simulink model "constraints_comparison_A_4D_v2_old"  (R2016a)
settings: Solver=ode4  StartTime=0.0  StopTime=10  FixedStep=0.0001  RelTol=1e-3
InitFcn:
  | clear
  | clc
undefined symbols (not defined in the file or in its folder): acm_aero_model, acm_T_N, breakpoints1, Cm0, Cmde, Cmq, dail, de, dele, drud, Fr_mp_1, Fr_mp_2, Fr_rp_1, Fr_rp_2, ini_acm_de_deg, ini_acm_p_deg_per_s, ini_acm_phi_deg, ini_acm_psi_deg, ini_acm_q_deg_per_s, ini_acm_r_deg_per_s, ini_acm_theta_deg, ini_cmp_de_deg, ini_rig_p_deg_per_s, ini_rig_phi_deg, ini_rig_psi_deg, ini_rig_q_deg_per_s, ini_rig_r_deg_per_s, ini_rig_theta_deg, K1_svo_acm, K1_svo_cmp, K2_svo_acm, K2_svo_cmp, La, Ma, max_defl_sat_acm, max_defl_sat_cmp, max_rate_sat, max_rate_sat_acm, max_rate_sat_cmp, Na, sigbuilder_block, simstop, windspeed, Xa, Ya, Za
libraries: aerolibconvert2 x117, simulink x42, aerolibtransform2 x19, vrlib x2
(part 2 of 6)

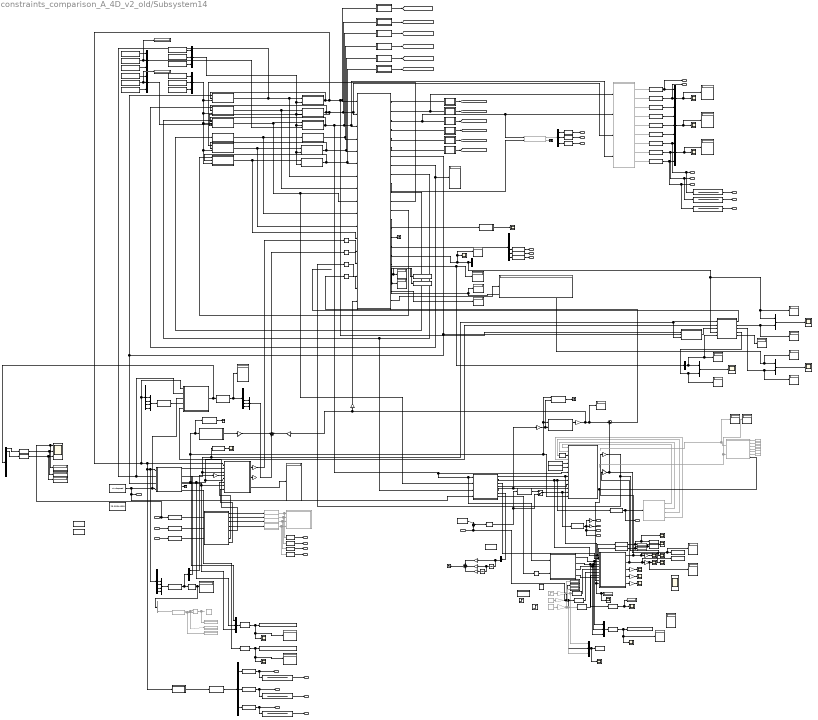
== system constraints_comparison_A_4D_v2_old/Subsystem14 ==
  note: yaw
  note: pitch
  note: roll
  note: Estimated reaction forces
  note: Simulation aircraft reaction forces
  note: Estimated laod cell reading
  note: Simulation load cell reading
  note: ALTITUDE CONTROL
  note: Estimated estimated load cell moment
  note: Simulation load cell moment
  ACM_de_c(deg) : Inport
  CMP_da_c(deg) : Inport  Port=2
  CMP_de_c(deg) : Inport  Port=3
  CMP_dr_c(deg) : Inport  Port=4
  Aerodynamics lookup : Subsystem  Commented=on
  Aerodynamics model: Hawk : MATLAB Function
      settings: MinAlgLoopOccurrences=on
  Aerodynamics model: compensator : MATLAB Function
      settings: MinAlgLoopOccurrences=on
  Aircraft acceleration body axis : MATLAB Function  Commented=on  TreatAsAtomicUnit=on
  Aircraft attitude relative to arm2 : MATLAB Function  Commented=on  TreatAsAtomicUnit=on
  Aircraft loads for load case loop : MATLAB Function  Commented=on
      settings: MinAlgLoopOccurrences=on
  Aircraft model vertical reaction force : Scope
  Aircraft_model_friction : MATLAB Function
      settings: MinAlgLoopOccurrences=on
  Angle Conversion{,1,3,6,8..12,14..26,29..34,37..38,40} (31 alike) : aerolibconvert2/Angle Conversion  IU=rad  OU=deg
  Angle Conversion{2,4,7,13,27..28,35,39} (8 alike) : aerolibconvert2/Angle Conversion  IU=deg  OU=rad
  Butterworth filter (cutoff frequency 10Hz) + differentiating{,1..5} (6 alike) : TransferFcn  Numerator=[1 0]  Denominator=[2.5330e-04 0.0225 1]
  CMP aero model : MATLABFcn  MATLABFcn=Cmp_aero_model
  Calculating rig pitch acceleration : MATLAB Function  TreatAsAtomicUnit=on
  Chirp Signal : simulink/Sources/Chirp Signal  Commented=on  f1=0.5  T=120  f2=3
  Chirp Signal1 : simulink/Sources/Chirp Signal  Commented=on  f1=0.5  T=120  f2=3
  Chirp Signal2 : simulink/Sources/Chirp Signal  f1=0.5  T=120  f2=3
  Comparing simulation aircraft reaction forces and estimated reaction forces : Scope
  Comparing simulation aircraft reaction forces and estimated reaction forces1 : Scope
  Comparing simulation load cell reading and estimated load cell reading : Scope
  Compensator friction : MATLAB Function
      settings: MinAlgLoopOccurrences=on
  Compensator servo model1 : Subsystem  Commented=on
  Compensator servo model2 : Subsystem  Commented=on
  Compensator servo model3 : Subsystem  Commented=on
  Compensator servo model4 : Subsystem  Commented=on
  Constant : Constant  Commented=on  Value=simstop
  Constant10 : Constant  Value=7.515637662
  Constant11 : Constant  Value=0
  Constant2 : Constant  Value=-7.308232274
  Constant3 : Constant  Value=14.34612797
  Cq_transpose_lc CHECK : Display
  Demux : Demux  Outputs=7
  Demux{1..3,5..6,12} (6 alike) : Demux  Outputs=3
  Demux10 : Demux  Outputs=11
  Demux4 : Demux  Commented=on  Outputs=3
  Demux7 : Demux  Outputs=6
  Demux8 : Demux  Outputs=7
  Demux9 : Demux  Outputs=6
  Derivative : Derivative
  Display{,2..3,5..6,8..14,18} (13 alike) : Display
  Display15 : Display  Commented=on
  Display16 : Display  Commented=on
  Display17 : Display  Commented=on
  Equations of Motion : MATLAB Function
      settings: MinAlgLoopOccurrences=on
  Extracting aircraft vertical reaction forces1 : MATLAB Function  TreatAsAtomicUnit=on
  Extracting position vector 1 : Subsystem
  Extracting position vector 2 : Subsystem
  "Extracting position vector 2 " : Subsystem
  Extracting position vector 3 : Subsystem
  Extracting position vector 4 : Subsystem
  Extracting position vector 5 : Subsystem
  F : Display
  FF : Display
  Fcn : Fcn  Expr=u/9.81
  Fcn1 : Fcn  Expr=u/9.81
  Fcn2 : Fcn  Expr=u/9.81
  Friction_estimate : Display
  Friction_moment : Display
  Gain{,3,6..7,11,14,28} (7 alike) : Gain  Gain=-1
  Gain{4,8..10,17,19..23,30} (11 alike) : Gain
  Gain12 : Gain  Gain=0
  Gain13 : Gain  Gain=0
  Gain24 : Gain  Commented=on  Gain=dail
  Gain25 : Gain  Commented=on  Gain=dele
  Gain27 : Gain  Commented=on  Gain=drud
  HHIRM : MATLAB Function
      settings: MinAlgLoopOccurrences=on
  Hawk servo model : Subsystem
  IC{1..4} (4 alike) : InitialCondition  Value=0
  Integrator : Integrator
  Integrator1 : Integrator
  L : Constant  Commented=on  Value=La
  Load cell reading to aircraft reaction forces : MATLAB Function  TreatAsAtomicUnit=on
  M : Display
  M1 : Constant  Commented=on  Value=Ma
  MATLAB Function1 : MATLAB Function  TreatAsAtomicUnit=on
  MATLAB Function10 : MATLAB Function  TreatAsAtomicUnit=on
  MATLAB Function2 : MATLAB Function  TreatAsAtomicUnit=on
  MATLAB Function3 : MATLAB Function
      settings: MinAlgLoopOccurrences=on
  MATLAB Function4 : MATLAB Function  TreatAsAtomicUnit=on
  MATLAB Function5 : MATLAB Function
      settings: MinAlgLoopOccurrences=on
  MATLAB Function6 : MATLAB Function  TreatAsAtomicUnit=on
  MATLAB Function7 : MATLAB Function
      settings: MinAlgLoopOccurrences=on
  MATLAB Function8 : MATLAB Function  TreatAsAtomicUnit=on
  MATLAB Function9 : MATLAB Function  TreatAsAtomicUnit=on
  MM : Display
  Manual Switch1 : ManualSwitch  CurrentSetting=0
  Mux{,2..4,7..10,12..13,15} (11 alike) : Mux  Inputs=3
  Mux1 : Mux  Inputs=2
  Mux11 : Mux
  Mux14 : Mux
  Mux5 : Mux  Inputs=2
  Mux6 : Mux  Inputs=2
  N : Constant  Commented=on  Value=Na
  Physical deflections to virtual compensator deflections : MATLAB Function  Commented=on  TreatAsAtomicUnit=on
  Quaternions to Rotation Angles : aerolibtransform2/Quaternions to Rotation Angles  rotationOrder=ZYX
  Quaternions to Rotation Angles1 : aerolibtransform2/Quaternions to Rotation Angles  rotationOrder=ZYX
  Quaternions to Rotation Angles2 : aerolibtransform2/Quaternions to Rotation Angles  rotationOrder=ZYX
  Relational Operator : RelationalOperator  Commented=on  OutDataTypeStr=boolean
  Relative angle from rotation matrix : Scope
  Rotation angles from rotation matrix (acm) : Scope
  Rotation angles from rotation matrix (arm) : Scope
  Scope{,1..8,10..13} (13 alike) : Scope
  Scope14 : Scope  NumInputPorts=3
  Scope9 : Scope  NumInputPorts=5
  Signal Builder : Subsystem  Tag=STV Subsys  LoadFcn=sigbuilder_block('load');  StartFcn=sigbuilder_block('start');  StopFcn=sigbuilder_block('stop');  ClipboardFcn=sigbuilder_block('clipboard');  mask(Sigbuilder block){}
      mask help: Simulink:masks:SigbuilderBlock_MD
      mask init:
      | if ~strcmp(get_param(bdroot(gcbh),'SimulationStatus'),'stopped') tuvar = sigbuilder_block('maskInit'); end
      settings: CopyFcn=sigbuilder_block('copy');  DeleteFcn=sigbuilder_block('delete');  ModelCloseFcn=sigbuilder_block('modelClose');  PreSaveFcn=sigbuilder_block('preSave');  PauseFcn=sigbuilder_block('pause');  ContinueFcn=sigbuilder_block('continue');  NameChangeFcn=sigbuilder_block('namechange');  OpenFcn=sigbuilder_block('open',[437.6 199.2 550.4 400 ]);  CloseFcn=sigbuilder_block('close');
      mask Display: plot(0, 0, 100, 100,[2, 2, 32, 32, 2], [68, 8, 8, 68, 68],[32, 2], [38, 38], [32, 19, 2],[53, 60, 44], [32, 17, 17, 2],[16, 16, 31, 31]);txt = getActiveGroup(gcbh);text(2, 100, txt,'verticalAlignment', 'top');
  Step : Step  Commented=on  Time=0.01  SampleTime=0
  Step2 : Step  SampleTime=0
  Step3 : Step  SampleTime=0
  Stop Simulation : Stop  Commented=on
  Subsystem : Subsystem
  Subsystem1 : Subsystem
  Subsystem10 : Subsystem
  Subsystem11 : Subsystem
  Subsystem12 : Subsystem
  Subsystem13 : Subsystem
  Subsystem2 : Subsystem
  Subsystem3 : Subsystem
  Subsystem4 : Subsystem
  Subsystem5 : Subsystem
  Subsystem6 : Subsystem
  Subsystem7 : Subsystem
  Subsystem8 : Subsystem
  Subsystem9 : Subsystem
  Sum2 : Sum  Inputs=|++
  Sum3 : Sum
  Sum5 : Sum  Inputs=+++
  Sum8 : Sum  Inputs=++-
  Terminator{,1..5} (6 alike) : Terminator
  To Workspace : ToWorkspace  VariableName=reaction_forces_lc_body_N  SaveFormat=Timeseries  SampleTime=-1
  To Workspace1 : ToWorkspace  VariableName=reaction_moments_lc_body_Nm  SaveFormat=Timeseries  SampleTime=-1
  To Workspace2 : ToWorkspace  VariableName=cs_deg  SaveFormat=Timeseries  SampleTime=-1
  To Workspace3 : ToWorkspace  VariableName=alpha_deg  SaveFormat=Timeseries  SampleTime=-1
  To Workspace4 : ToWorkspace  VariableName=beta_deg  SaveFormat=Timeseries  SampleTime=-1
  To Workspace5 : ToWorkspace  VariableName=aero_forces_N  SaveFormat=Timeseries  SampleTime=-1
  To Workspace6 : ToWorkspace  VariableName=aero_moments_Nm  SaveFormat=Timeseries  SampleTime=-1
  To Workspace7 : ToWorkspace  VariableName=wind_axes_rotation_rates_degpers  SaveFormat=Timeseries  SampleTime=-1
  To Workspace8 : ToWorkspace  VariableName=inertial_axes_CMP_rotation_rates_degpers  SaveFormat=Timeseries  SampleTime=-1
  To Workspace9 : ToWorkspace  VariableName=inertial_axes_CMP_rotation_accelerations_degperspers  SaveFormat=Timeseries  SampleTime=-1
  V{,1..3} (4 alike) : Display
  Virtual compensator deflections to physical deflections : MATLAB Function  TreatAsAtomicUnit=on
  Wind axes angular rates calculation : MATLAB Function
      settings: MinAlgLoopOccurrences=on
  Wind tunnel velocity : Constant  Value=windspeed
  Wind tunnel velocity1 : Constant  Value=25.09344509
  X : Constant  Commented=on  Value=Xa
  Y : Constant  Commented=on  Value=Ya
  Z : Constant  Commented=on  Value=Za
  acm_T_N : Constant  Value=acm_T_N
  acm_aero_model : Constant  Value=acm_aero_model
  aircraft_cell_reaction_forces : Display
  aircraft_cell_reaction_moments : Display
  alpha : Display
  alpha1 : Display
  alpha2 : Scope
  beta2 : Scope
  ini_acm_q_deg_per_s : Constant  Value=ini_acm_q_deg_per_s
  ini_acm_q_deg_per_s2 : Constant  Value=ini_acm_p_deg_per_s
  ini_acm_q_deg_per_s3 : Constant  Value=ini_acm_r_deg_per_s
  ini_acm_theta_deg : Constant  Value=ini_acm_theta_deg
  ini_acm_theta_deg2 : Constant  Value=ini_acm_phi_deg
  ini_acm_theta_deg3 : Constant  Value=ini_acm_psi_deg
  ini_rig_theta_deg : Constant  Value=ini_rig_theta_deg
  ini_rig_theta_deg2 : Constant  Value=ini_rig_psi_deg
  ini_rig_theta_deg3 : Constant  Value=ini_rig_phi_deg
  ini_rig_theta_deg_per_s : Constant  Value=ini_rig_q_deg_per_s
  ini_rig_theta_deg_per_s2 : Constant  Value=ini_rig_p_deg_per_s
  ini_rig_theta_deg_per_s3 : Constant  Value=ini_rig_r_deg_per_s
  load_cell_reaction_forces{,2..8} (8 alike) : Display
  load_cell_reaction_forces_body : Display
  load_cell_reaction_moments : Display
  load_cell_reaction_moments_body : Display
  q : Display
  q1 : Display
  rates : Display
  theta_rig : Scope
  z_reaction_force : Scope
  GX(deg/s) : Outport
  GY(deg/s) : Outport  Port=2
  GZ(deg/s) : Outport  Port=3
  Nx : Outport  Port=4
  Ny : Outport  Port=5
  Nz : Outport  Port=6
  ACM_roll(deg) : Outport  Port=7
  ACM_rollrate(deg/s) : Outport  Port=8
  ACM_pitch(deg) : Outport  Port=9
  ACM_pitchrate(deg/s) : Outport  Port=10
  ACM_yaw(deg) : Outport  Port=11
  ACM_yawrate(deg/s) : Outport  Port=12
  RIG_roll(deg) : Outport  Port=13
  RIG_rollrate(deg/s) : Outport  Port=14
  RIG_pitch(deg) : Outport  Port=15
  RIG_pitchrate(deg/s) : Outport  Port=16
  RIG_yaw(deg) : Outport  Port=17
  RIG_yawrate(deg/s) : Outport  Port=18
  delta_el_c(deg) : Outport  Port=19
  delta_el(deg) : Outport  Port=20
  delta_er_c(deg) : Outport  Port=21
  delta_er(deg) : Outport  Port=22
  delta_cmp1(deg) : Outport  Port=23
  delta_cmp2(deg) : Outport  Port=24
  delta_cmp3(deg) : Outport  Port=25
  delta_cmp4(deg) : Outport  Port=26
  wind speed(m/s) : Outport  Port=27
  AoA(deg) : Outport  Port=28
  roll_ac(deg) : Outport  Port=29
  pitch_ac(deg) : Outport  Port=30
  tag scope: animation_acm_rotation=global, animation_acm_translation=global, animation_arm_rotation=global, animation_arm_translation=global, animation_cmp_rotation=global, animation_cmp_translation=global, animation_link_rotation=global, animation_link_translation=global, animation_load_cell_rotation=global, animation_load_cell_translation=global, animation_mass_rotation=global, animation_mass_translation=global
  wires:
  Equations of Motion/2(Ar) -> Aircraft attitude relative to arm2/1(Ar), MATLAB Function1/1(A2)
  Equations of Motion/8(qr_dot_dot) -> Subsystem2/1(In1), load_cell_reaction_forces8/1
  Subsystem2/1(Out1) -> Equations of Motion/8(qr_dot), Subsystem3/1(In1)
  Angle Conversion2/1 -> Hawk servo model/1(Command), Manual Switch1/2
  Sum3/1 -> Angle Conversion2/1  "Hawk elevator (deg)"
  Equations of Motion/11(qm_dot_dot) -> Subsystem8/1(In1)
  Subsystem8/1(Out1) -> Equations of Motion/10(qm_dot), Subsystem9/1(In1)
  Subsystem9/1(Out1) -> Extracting position vector 4/1(In1), Equations of Motion/4(qm)
  Equations of Motion/4(Am) -> MATLAB Function8/1(A3)
  Compensator friction/1(Fr_rp) -> Gain12/1
  Extracting aircraft vertical reaction forces1/1(RF_a) -> Aircraft model vertical reaction force/1
  Gain13/1 -> Friction_moment/1, Sum2/1, Gain30/1, Gain3/1  "Friction moment"
  Gain30/1 -> Sum8/3
  Gain20/1 -> Subsystem6/2(theta_dot_mp), Aircraft_model_friction/2(theta_dot_mp)
  Equations of Motion/14(RF) -> Extracting aircraft vertical reaction forces1/1(RF)
  Angle Conversion1/1 -> AoA(deg)/1, Aerodynamics lookup/1(Alpha (deg))  "Hawk alpha (deg)"
  MATLAB Function4/1(q2) -> Quaternions to Rotation Angles/1
  Quaternions to Rotation Angles/1 -> Demux3/1
  Demux3/2 -> Angle Conversion9/1
  Aircraft acceleration body axis/1(qa_dot_dot3) -> Demux5/1
  Integrator/1 -> Integrator1/1, Gain/1
  Demux6/3 -> Gain7/1, Integrator/1
  Gain/1 -> Sum5/2
  Integrator1/1 -> Gain6/1
  Gain6/1 -> Sum5/3
  Gain7/1 -> Sum5/1
  Demux3/1 -> Angle Conversion8/1
  Butterworth filter (cutoff frequency 10Hz) + differentiating/1 -> RIG_rollrate(deg/s)/1
  Butterworth filter (cutoff frequency 10Hz) + differentiating2/1 -> RIG_yawrate(deg/s)/1
  Demux3/3 -> Angle Conversion10/1
  Angle Conversion8/1 -> RIG_roll(deg)/1, Butterworth filter (cutoff frequency 10Hz) + differentiating/1
  Angle Conversion9/1 -> Butterworth filter (cutoff frequency 10Hz) + differentiating1/1, RIG_pitch(deg)/1
  Angle Conversion10/1 -> RIG_yaw(deg)/1, Butterworth filter (cutoff frequency 10Hz) + differentiating2/1
  Demux5/1 -> Fcn/1
  Demux5/2 -> Fcn1/1
  Demux5/3 -> Fcn2/1
  Equations of Motion/16(qa_dot2) -> Demux7/1
  Demux7/4 -> Angle Conversion/1
  Demux7/5 -> Angle Conversion11/1
  Demux7/6 -> Angle Conversion12/1
  Fcn/1 -> Nx/1
  Fcn1/1 -> Ny/1
  Fcn2/1 -> Nz/1
  Angle Conversion/1 -> GX(deg/s)/1
  Angle Conversion11/1 -> GY(deg/s)/1
  Angle Conversion12/1 -> GZ(deg/s)/1
  Subsystem3/1(Out1) -> Subsystem2/2(q), Subsystem4/5(qr), "Extracting position vector 2 "/1(In1), Equations of Motion/2(qr), Aircraft attitude relative to arm2/3(qr)
  Equations of Motion/3(Aa) -> MATLAB Function6/1(A3), Aircraft acceleration body axis/1(Aa), Aircraft attitude relative to arm2/2(Aa)
  Mux2/1 -> Relative angle from rotation matrix/1, Display/1
  Aircraft attitude relative to arm2/7(phi_relative) -> Angle Conversion16/1
  Aircraft attitude relative to arm2/9(psi_relative) -> Angle Conversion18/1
  Angle Conversion18/1 -> Butterworth filter (cutoff frequency 10Hz) + differentiating5/1, ACM_yaw(deg)/1, Mux2/3  "Yaw"
  Angle Conversion17/1 -> Mux2/2, Butterworth filter (cutoff frequency 10Hz) + differentiating4/1, ACM_pitch(deg)/1  "Pitch"
  Angle Conversion16/1 -> ACM_roll(deg)/1, Butterworth filter (cutoff frequency 10Hz) + differentiating3/1, Mux2/1  "Roll"
  Mux3/1 -> Display2/1, Rotation angles from rotation matrix (acm)/1
  Angle Conversion21/1 -> Mux3/3  "Yaw"
  Angle Conversion20/1 -> pitch_ac(deg)/1, Mux3/2  "Pitch"
  Angle Conversion19/1 -> roll_ac(deg)/1, Mux3/1  "Roll"
  Aircraft attitude relative to arm2/1(phi_acm) -> Angle Conversion19/1
  Aircraft attitude relative to arm2/2(theta_acm) -> Angle Conversion20/1
  Aircraft attitude relative to arm2/3(psi_acm) -> Angle Conversion21/1
  Mux4/1 -> Rotation angles from rotation matrix (arm)/1, Display3/1
  Angle Conversion24/1 -> Mux4/3  "Yaw"
  Angle Conversion23/1 -> Mux4/2  "Pitch"
  Angle Conversion22/1 -> Mux4/1  "Roll"
  Aircraft attitude relative to arm2/4(phi_arm) -> Angle Conversion22/1
  Aircraft attitude relative to arm2/5(theta_arm) -> Angle Conversion23/1
  Aircraft attitude relative to arm2/6(psi_arm) -> Angle Conversion24/1
  Butterworth filter (cutoff frequency 10Hz) + differentiating3/1 -> ACM_rollrate(deg/s)/1
  Butterworth filter (cutoff frequency 10Hz) + differentiating4/1 -> ACM_pitchrate(deg/s)/1
  Butterworth filter (cutoff frequency 10Hz) + differentiating5/1 -> ACM_yawrate(deg/s)/1
  CMP_da_c(deg)/1 -> Display12/1, Scope14/1, Angle Conversion35/1  "input (deg)"
  CMP_dr_c(deg)/1 -> Angle Conversion39/1
  Angle Conversion6/1 -> Gain11/1, Gain14/1, delta_er(deg)/1, delta_er_c(deg)/1
  Virtual compensator deflections to physical deflections/1(servo1) -> Compensator servo model1/1(Command)
  Virtual compensator deflections to physical deflections/2(servo2) -> Compensator servo model2/1(Command)
  Virtual compensator deflections to physical deflections/3(servo3) -> Compensator servo model3/1(Command)
  Virtual compensator deflections to physical deflections/4(servo4) -> Compensator servo model4/1(Command)
  Angle Conversion4/1 -> Aerodynamics model: Hawk/3(de)
  Aerodynamics lookup/1(Cm0) -> Aerodynamics model: Hawk/1(Cm0)
  Aerodynamics lookup/2(Cmde) -> Aerodynamics model: Hawk/2(Cmde)
  Aerodynamics lookup/3(de_deg) -> Angle Conversion4/1
  Aerodynamics lookup/4(Cmq) -> Aerodynamics model: Hawk/4(Cmq)
  Angle Conversion14/1 -> delta_cmp1(deg)/1
  Angle Conversion15/1 -> delta_cmp2(deg)/1
  Angle Conversion25/1 -> delta_cmp3(deg)/1
  Angle Conversion26/1 -> delta_cmp4(deg)/1
  MATLAB Function2/1(A11) -> [animation_cmp_rotation]
  MATLAB Function1/1(A22) -> [animation_arm_rotation]
  MATLAB Function6/1(A33) -> [animation_acm_rotation]
  MATLAB Function8/1(A33) -> [animation_mass_rotation]
  Extracting position vector 1/1(Out1) -> [animation_cmp_translation]
  "Extracting position vector 2 "/1(Out1) -> [animation_arm_translation]
  Extracting position vector 3/1(Out1) -> [animation_acm_translation]
  Extracting position vector 4/1(Out1) -> [animation_mass_translation]
  Compensator servo model1/1(Response) -> Angle Conversion14/1, Physical deflections to virtual compensator deflections/1(servo1)
  Compensator servo model2/1(Response) -> Angle Conversion15/1, Physical deflections to virtual compensator deflections/2(servo2)
  Compensator servo model3/1(Response) -> Angle Conversion25/1, Physical deflections to virtual compensator deflections/3(servo3)
  Compensator servo model4/1(Response) -> Angle Conversion26/1, Physical deflections to virtual compensator deflections/4(servo4)
  Equations of Motion/1(Ac) -> MATLAB Function2/1(A1)
  Manual Switch1/1 -> Angle Conversion6/1, Aerodynamics model: Hawk/12(eta)
  Virtual compensator deflections to physical deflections/7(de_cmp2) -> Aerodynamics model: compensator/6(eta)
  MATLAB Function7/1(V_t) -> Aerodynamics model: compensator/2(V_t)
  MATLAB Function3/1(V0) -> HHIRM/11(V), Scope6/1, V/1, Aerodynamics model: Hawk/8(V0)
  MATLAB Function3/2(alpha) -> Angle Conversion3/1, HHIRM/1(alpha), Angle Conversion1/1, Aerodynamics model: Hawk/9(alpha)
  MATLAB Function3/4(w_dot) -> Aerodynamics model: Hawk/10(w_dot)
  MATLAB Function3/5(q) -> Gain20/1, Aerodynamics model: Hawk/11(q)
  MATLAB Function3/6(Va) -> Demux6/1
  Aerodynamics model: compensator/1(F_c) -> Gain4/1
  Aerodynamics model: compensator/2(M_dash_c) -> Gain8/1
  Gain12/1 -> Sum8/1
  Equations of Motion/10(qa_dot_dot2) -> Aircraft acceleration body axis/2(qa_dot_dot2)
  Aircraft attitude relative to arm2/8(theta_relative) -> Angle Conversion17/1
  Aircraft_model_friction/1(Fr_mp) -> Gain13/1
  Mux15/1 -> Sum8/2
  Hawk servo model/1(Response) -> Manual Switch1/1
  Gain4/1 -> IC1/1
  Sum8/1 -> IC2/1
  Gain10/1 -> Scope5/1, IC3/1
  Sum2/1 -> IC4/1
  Subsystem5/1(Out1) -> Extracting position vector 3/1(In1), Equations of Motion/3(qa), Aircraft attitude relative to arm2/4(qa), Wind axes angular rates calculation/1(qa), MATLAB Function3/1(qa), Aerodynamics model: Hawk/7(qa), Subsystem4/2(qa)
  Subsystem4/1(Out1) -> Subsystem5/1(In1), MATLAB Function3/2(qa_dot), Equations of Motion/9(qa_dot)
  Equations of Motion/9(qa_dot_dot) -> Subsystem4/1(In1), MATLAB Function3/3(qa_dot_dot)
  IC1/1 -> Equations of Motion/13(F_c)
  IC2/1 -> Equations of Motion/14(M_dash_c)
  IC3/1 -> Equations of Motion/15(F_a)
  IC4/1 -> Equations of Motion/16(M_dash_a)
  Mux8/1 -> Subsystem1/2(rig attitude), Subsystem3/2(rig attitude), Subsystem5/2(rig attitude), Subsystem11/2(rig attitude), Subsystem13/2(rig attitude)
  Mux/1 -> Subsystem5/3(acm attitude)
  Gain11/1 -> delta_el_c(deg)/1
  Gain14/1 -> delta_el(deg)/1
  Angle Conversion13/1 -> Virtual compensator deflections to physical deflections/2(de_cmp)
  CMP_de_c(deg)/1 -> Angle Conversion13/1  "Compensator elevator (deg)"
  Mux13/1 -> Subsystem4/3(rotation_rates), Subsystem12/3(rotation_rates), Subsystem10/3(rotation_rates), Subsystem2/3(rotation_rates), Subsystem/3(rotation_rates)
  Mux7/1 -> Subsystem4/4(angular rates (body))
  Subsystem10/1(Out1) -> Equations of Motion/11(qlc_dot), Subsystem11/1(In1)
  Equations of Motion/12(qlc_dot_dot) -> Subsystem10/1(In1)
  Subsystem13/1(Out1) -> Subsystem12/2(q), Equations of Motion/6(ql), Extracting position vector 5/1(In1)
  Equations of Motion/13(ql_dot_dot) -> Subsystem12/1(In1)
  Extracting position vector 2/1(Out1) -> [animation_load_cell_translation]
  Extracting position vector 5/1(Out1) -> [animation_link_translation]
  Subsystem11/1(Out1) -> Subsystem10/2(q), Extracting position vector 2/1(In1), Equations of Motion/5(qlc)
  MATLAB Function9/1(A33) -> [animation_load_cell_rotation]
  MATLAB Function10/1(A33) -> [animation_link_rotation]
  Equations of Motion/5(Alc) -> MATLAB Function9/1(A3)
  Equations of Motion/6(Al) -> MATLAB Function10/1(A3)
  Subsystem12/1(Out1) -> Equations of Motion/12(ql_dot), Subsystem13/1(In1)
  Aircraft acceleration body axis/2(nz) -> Terminator/1
  Equations of Motion/15(RF_arm) -> Terminator1/1
  MATLAB Function7/6(Vc) -> Terminator2/1
  Subsystem7/1(Fr_mp) -> Terminator3/1
  Subsystem6/1(Fr_mp) -> Terminator4/1
  Sum5/1 -> Terminator5/1  "de_acm"
  Constant11/1 -> Sum3/1
  acm_T_N/1 -> Aerodynamics model: Hawk/5(T)
  acm_aero_model/1 -> Aerodynamics model: Hawk/6(acm_aero_model)
  Butterworth filter (cutoff frequency 10Hz) + differentiating1/1 -> RIG_pitchrate(deg/s)/1
  Wind tunnel velocity/1 -> wind speed(m/s)/1, MATLAB Function3/4(Vt), MATLAB Function5/3(Vt), MATLAB Function7/4(Vt)
  Equations of Motion/17(reaction_forces_lc) -> z_reaction_force/1, load_cell_reaction_forces/1, Load cell reading to aircraft reaction forces/4(R_reading), load_cell_reaction_forces2/1, Mux1/1, Demux12/1
  Equations of Motion/22(reaction_moments_a) -> aircraft_cell_reaction_moments/1
  Demux2/2 -> Angle Conversion31/1, Calculating rig pitch acceleration/3(theta_r), Load cell reading to aircraft reaction forces/1(theta_r), Aerodynamics model: compensator/3(alpha)
  Load cell reading to aircraft reaction forces/1(F_acm) -> ?
  Mux1/1 -> Comparing simulation load cell reading and estimated load cell reading/1
  Load cell reading to aircraft reaction forces/2(R) -> load_cell_reaction_forces3/1, Mux1/2
  Calculating rig pitch acceleration/1(theta_r_dot_dot) -> Load cell reading to aircraft reaction forces/3(theta_r_dot_dot)
  Mux5/1 -> Comparing simulation aircraft reaction forces and estimated reaction forces/1
  Load cell reading to aircraft reaction forces/3(R_a) -> load_cell_reaction_forces5/1, Mux5/2
  Equations of Motion/21(reaction_forces_a) -> aircraft_cell_reaction_forces/1, load_cell_reaction_forces4/1, Mux5/1
  Mux6/1 -> Comparing simulation aircraft reaction forces and estimated reaction forces1/1
  Load cell reading to aircraft reaction forces/4(M) -> load_cell_reaction_forces7/1, Mux6/2
  Equations of Motion/18(reaction_moments_lc) -> Demux1/1, load_cell_reaction_moments/1
  Demux1/2 -> Mux6/1, Load cell reading to aircraft reaction forces/5(M_reading), load_cell_reaction_forces6/1
  Gain3/1 -> Equations of Motion/17(M_dash_l)
  Load cell reading to aircraft reaction forces/5(Friction_estimate) -> Friction_estimate/1
  MATLAB Function3/7(qa_wind) -> Derivative/1
  Derivative/1 -> Wind axes angular rates calculation/2(qa_wind_dot)
  Wind axes angular rates calculation/1(p) -> Mux10/1, HHIRM/3(p)
  Wind axes angular rates calculation/3(r) -> Mux10/3, HHIRM/5(r)
  MATLAB Function3/3(beta) -> Angle Conversion30/1, HHIRM/2(beta)
  Gain17/1 -> Scope/1
  HHIRM/5(CZ) -> Gain17/1
  Wind axes angular rates calculation/4(A_b2w) -> HHIRM/9(A_b2w)
  Gain19/1 -> Scope1/1
  HHIRM/3(CX) -> Gain19/1
  Gain21/1 -> Scope2/1
  HHIRM/4(CY) -> Gain21/1
  Gain22/1 -> Scope3/1
  Gain23/1 -> M/1, Scope4/1
  ini_acm_theta_deg3/1 -> Mux/1
  ini_acm_theta_deg/1 -> Display5/1, Mux/2
  ini_acm_theta_deg2/1 -> Mux/3
  ini_acm_q_deg_per_s2/1 -> Mux7/1
  ini_acm_q_deg_per_s3/1 -> Mux7/3
  ini_rig_theta_deg/1 -> Mux8/2
  ini_rig_theta_deg2/1 -> Mux8/1
  ini_rig_theta_deg3/1 -> Mux8/3
  Angle Conversion3/1 -> alpha2/1, To Workspace3/1, alpha/1
  Equations of Motion/19(reaction_forces_lc_body) -> To Workspace/1, load_cell_reaction_forces_body/1
  Equations of Motion/20(reaction_moments_lc_body) -> load_cell_reaction_moments_body/1, To Workspace1/1
  Step/1 -> Gain24/1
  Chirp Signal/1 -> Gain25/1
  Chirp Signal1/1 -> Gain27/1
  Gain24/1 -> V1/1, Mux9/1, Angle Conversion7/1
  ACM_de_c(deg)/1 -> Angle Conversion27/1, Mux9/2, V2/1, Sum3/2
  Angle Conversion7/1 -> HHIRM/6(dail)
  Angle Conversion27/1 -> HHIRM/7(dele)
  Angle Conversion28/1 -> HHIRM/8(drud)
  Wind axes angular rates calculation/2(q) -> Angle Conversion29/1, Mux10/2, HHIRM/4(q)
  Angle Conversion29/1 -> q/1, Scope7/1
  Gain27/1 -> V3/1, Mux9/3, Angle Conversion28/1
  Gain9/1 -> Scope8/1, Sum2/2
  HHIRM/2(M_dash_a) -> Gain9/1, To Workspace6/1, Gain23/1
  HHIRM/1(Fa) -> Gain10/1, F/1, To Workspace5/1, Gain22/1
  Mux9/1 -> Scope10/1, To Workspace2/1
  Angle Conversion30/1 -> beta2/1, To Workspace4/1, alpha1/1
  Angle Conversion31/1 -> theta_rig/1
  Mux10/1 -> Angle Conversion32/1
  Angle Conversion32/1 -> To Workspace7/1, rates/1, Scope11/1
  Quaternions to Rotation Angles1/1 -> Demux2/1, Angle Conversion33/1
  Angle Conversion33/1 -> Demux4/1, Display6/1
  Demux/7 -> Mux11/4
  Demux/6 -> Mux11/3
  Demux/5 -> Mux11/2
  Demux/4 -> Mux11/1
  Mux11/1 -> Quaternions to Rotation Angles1/1
  MATLAB Function7/3(p) -> Mux12/1
  MATLAB Function7/5(r) -> Aerodynamics model: compensator/7(r), Mux12/3
  MATLAB Function7/4(q) -> Aerodynamics model: Hawk/13(q_rig), Subsystem6/1(theta_dot_rp), Aircraft_model_friction/1(theta_dot_rp), Subsystem7/1(theta_dot_rp), Compensator friction/1(theta_dot_rp), Mux12/2, Load cell reading to aircraft reaction forces/2(theta_r_dot), Aerodynamics model: compensator/5(q)
  Mux12/1 -> Angle Conversion34/1
  Equations of Motion/7(qc_dot_dot) -> Subsystem/1(In1), MATLAB Function7/3(qc_dot_dot), Calculating rig pitch acceleration/2(qc_dot_dot)
  Subsystem/1(Out1) -> MATLAB Function7/2(qc_dot), MATLAB Function5/2(qc_dot), Equations of Motion/7(qc_dot), Subsystem1/1(In1)
  Angle Conversion37/1 -> Scope13/1, Display11/1, To Workspace9/1
  MATLAB Function7/7(omega_dashc_dot) -> Angle Conversion37/1
  ini_rig_theta_deg_per_s/1 -> Mux13/2
  ini_rig_theta_deg_per_s3/1 -> Mux13/3
  ini_rig_theta_deg_per_s2/1 -> Mux13/1
  Angle Conversion35/1 -> Virtual compensator deflections to physical deflections/1(da_cmp)
  Angle Conversion39/1 -> Virtual compensator deflections to physical deflections/3(dr_cmp)
  ini_acm_q_deg_per_s/1 -> Display8/1, Mux7/2
  Angle Conversion34/1 -> To Workspace8/1, Display9/1, Scope12/1
  Constant/1 -> Display17/1, Relational Operator/2
  Demux8/7 -> Mux14/4
  Demux8/6 -> Mux14/3
  Demux8/5 -> Mux14/2
  Demux8/4 -> Mux14/1
  Mux14/1 -> Quaternions to Rotation Angles2/1
  Subsystem1/1(Out1) -> Subsystem/2(q), Calculating rig pitch acceleration/1(qc), Extracting position vector 1/1(In1), Equations of Motion/1(qc), Aerodynamics model: compensator/1(qc), MATLAB Function4/1(q1), Demux/1, MATLAB Function7/1(qc), MATLAB Function5/1(qc), Demux8/1
  Quaternions to Rotation Angles2/1 -> MATLAB Function5/4(rotation_angles)
  MATLAB Function5/1(input) -> Demux10/1, CMP aero model/1
  Virtual compensator deflections to physical deflections/5(s2) -> MATLAB Function5/5(s)
  CMP aero model/1 -> Demux9/1, Display10/1
  Demux9/6 -> Mux15/3
  Demux9/5 -> Mux15/2
  Demux9/4 -> Mux15/1
  Demux10/1 -> Angle Conversion38/1
  Demux10/2 -> Angle Conversion40/1
  Angle Conversion38/1 -> Display13/1, Scope14/2  "phi (deg)"
  Angle Conversion40/1 -> Display14/1, Scope14/3  "p (deg/s)"
  Relational Operator/1 -> Display15/1
  Demux4/3 -> Display16/1, Relational Operator/1
  Aerodynamics model: Hawk/3(Aa) -> Aircraft loads for load case loop/7(A_b2i), HHIRM/10(A_b2i)
  Aircraft loads for load case loop/1(Fa) -> FF/1
  X/1 -> Aircraft loads for load case loop/1(X)
  Y/1 -> Aircraft loads for load case loop/2(Y)
  Z/1 -> Aircraft loads for load case loop/3(Z)
  L/1 -> Aircraft loads for load case loop/4(L)
  M1/1 -> Aircraft loads for load case loop/5(M)
  N/1 -> Aircraft loads for load case loop/6(N)
  Aircraft loads for load case loop/2(M_dash_a) -> MM/1
  Equations of Motion/23(Cq_transpose_lc_reaction) -> Cq_transpose_lc CHECK/1
  Gain28/1 -> Aerodynamics model: compensator/4(beta)
  Demux2/1 -> Gain28/1
  Virtual compensator deflections to physical deflections/8(dr_cmp2) -> Aerodynamics model: compensator/8(rudd)
  Aerodynamics model: compensator/3(extra) -> Display18/1

== system constraints_comparison_A_4D_v2_old/Trimmer ==
  qa : Inport
  Angle Conversion1 : aerolibconvert2/Angle Conversion  IU=rad  OU=deg
  Angle Conversion2 : aerolibconvert2/Angle Conversion  IU=rad  OU=deg
  Angle Conversion3 : aerolibconvert2/Angle Conversion  IU=rad  OU=deg
  Gain{,1..3} (4 alike) : Gain
  Mux : Mux  Inputs=3
  Trimming controller : Subsystem
  dail : Display
  dele : Display
  drud : Display
  thrust : Display
  cs_response (rad) : Outport
  thrust (N) : Outport  Port=2
  wires:
  Mux/1 -> cs_response (rad)/1
  Gain/1 -> Mux/1, Angle Conversion1/1  "dail"
  Gain3/1 -> Mux/2, Angle Conversion2/1  "dele"
  Gain1/1 -> Mux/3, Angle Conversion3/1  "drud"
  Trimming controller/2(dail) -> Gain/1
  Trimming controller/3(dele) -> Gain3/1
  Trimming controller/4(drud) -> Gain1/1
  Angle Conversion1/1 -> dail/1
  Angle Conversion2/1 -> dele/1
  Angle Conversion3/1 -> drud/1
  Trimming controller/1(thrust) -> Gain2/1
  Gain2/1 -> thrust (N)/1, thrust/1
  qa/1 -> Trimming controller/1(qa)

== system constraints_comparison_A_4D_v2_old/Control surface input/1) Short period ==
  note: Pulse width: 0.25s	0.1s		0.1s 	0.05s
      | Amplitude:	0.5deg	1.0deg	5.0deg	5.0deg
  Angle Conversion : aerolibconvert2/Angle Conversion  IU=deg  OU=rad
  Angle Conversion1 : aerolibconvert2/Angle Conversion  IU=deg  OU=rad
  Angle Conversion2 : aerolibconvert2/Angle Conversion  IU=deg  OU=rad
  Constant : Constant  Value=0
  Constant1 : Constant  Value=0
  Gain : Gain  Gain=2
  Mux : Mux  Inputs=3
  Signal Builder : Subsystem  Tag=STV Subsys  LoadFcn=sigbuilder_block('load');  StartFcn=sigbuilder_block('start');  StopFcn=sigbuilder_block('stop');  ClipboardFcn=sigbuilder_block('clipboard');  mask(Sigbuilder block){}
      mask help: Simulink:masks:SigbuilderBlock_MD
      mask init:
      | if ~strcmp(get_param(bdroot(gcbh),'SimulationStatus'),'stopped') tuvar = sigbuilder_block('maskInit'); end
      settings: CopyFcn=sigbuilder_block('copy');  DeleteFcn=sigbuilder_block('delete');  ModelCloseFcn=sigbuilder_block('modelClose');  PreSaveFcn=sigbuilder_block('preSave');  PauseFcn=sigbuilder_block('pause');  ContinueFcn=sigbuilder_block('continue');  NameChangeFcn=sigbuilder_block('namechange');  OpenFcn=sigbuilder_block('open',[168.75 4.5 1109.25 600.75 ]);  CloseFcn=sigbuilder_block('close');
      mask Display: plot(0, 0, 100, 100,[2, 2, 32, 32, 2], [68, 8, 8, 68, 68],[32, 2], [38, 38], [32, 19, 2],[53, 60, 44], [32, 17, 17, 2],[16, 16, 31, 31]);txt = getActiveGroup(gcbh);text(2, 100, txt,'verticalAlignment', 'top');
  Sum : Sum  Inputs=++|
  Sum1 : Sum  Inputs=++|
  Sum2 : Sum  Inputs=++|
  dail_ini : Constant  Value=0
  dele_ini : Constant  Value=-1.22537
  dele_ini1 : Constant  Value=-1.225
  drud_ini : Constant  Value=0
  cs_command (rad) : Outport
  wires:
  Angle Conversion2/1 -> Mux/3  "drud"
  Angle Conversion1/1 -> Mux/2  "dele"
  Angle Conversion/1 -> Mux/1  "dail"
  Mux/1 -> cs_command (rad)/1
  Signal Builder/1(Signal 1) -> Gain/1
  Constant/1 -> Sum/2
  Constant1/1 -> Sum2/2
  Gain/1 -> Sum1/2
  dail_ini/1 -> Sum/1
  dele_ini/1 -> Sum1/1
  drud_ini/1 -> Sum2/1
  Sum/1 -> Angle Conversion/1
  Sum1/1 -> Angle Conversion1/1
  Sum2/1 -> Angle Conversion2/1

== system constraints_comparison_A_4D_v2_old/Control surface input/2) Phugoid ==
  Angle Conversion : aerolibconvert2/Angle Conversion  IU=deg  OU=rad
  Angle Conversion1 : aerolibconvert2/Angle Conversion  IU=deg  OU=rad
  Angle Conversion2 : aerolibconvert2/Angle Conversion  IU=deg  OU=rad
  Constant : Constant  Value=0
  Constant1 : Constant  Value=0
  Gain : Gain
  Mux : Mux  Inputs=3
  Signal Builder : Subsystem  Tag=STV Subsys  LoadFcn=sigbuilder_block('load');  StartFcn=sigbuilder_block('start');  StopFcn=sigbuilder_block('stop');  ClipboardFcn=sigbuilder_block('clipboard');  mask(Sigbuilder block){}
      mask help: Simulink:masks:SigbuilderBlock_MD
      mask init:
      | if ~strcmp(get_param(bdroot(gcbh),'SimulationStatus'),'stopped') tuvar = sigbuilder_block('maskInit'); end
      settings: CopyFcn=sigbuilder_block('copy');  DeleteFcn=sigbuilder_block('delete');  ModelCloseFcn=sigbuilder_block('modelClose');  PreSaveFcn=sigbuilder_block('preSave');  PauseFcn=sigbuilder_block('pause');  ContinueFcn=sigbuilder_block('continue');  NameChangeFcn=sigbuilder_block('namechange');  OpenFcn=sigbuilder_block('open',[6 42.75 1428 641.25 ]);  CloseFcn=sigbuilder_block('close');
      mask Display: plot(0, 0, 100, 100,[2, 2, 32, 32, 2], [68, 8, 8, 68, 68],[32, 2], [38, 38], [32, 19, 2],[53, 60, 44], [32, 17, 17, 2],[16, 16, 31, 31]);txt = getActiveGroup(gcbh);text(2, 100, txt,'verticalAlignment', 'top');
  cs_command (rad) : Outport
  wires:
  Angle Conversion2/1 -> Mux/3  "drud"
  Angle Conversion1/1 -> Mux/2  "dele"
  Angle Conversion/1 -> Mux/1  "dail"
  Mux/1 -> cs_command (rad)/1
  Constant/1 -> Angle Conversion/1
  Constant1/1 -> Angle Conversion2/1
  Signal Builder/1(Signal 1) -> Gain/1
  Gain/1 -> Angle Conversion1/1

== system constraints_comparison_A_4D_v2_old/Control surface input/3) Roll subsidence ==
  note: Trim (wings level):
      | T = 2.037 N
      | dail = 0 deg
      | dele = -1.225 deg
      | drud = 0 deg
      | phi = 0 deg
      | theta = 1.612 deg
      | psi = 0 deg
      |
      | Trim (phi = -15 deg):
      | T = 2.225 N
      | dail = -30.39 deg
      | dele = -1.382 deg
      | drud = -36.89 deg
      | phi = -15.01 deg
      | theta = 5.134 deg
      | psi = 11.95 deg
      |
      | Trim (phi = -10 deg):
      | T = 2.026 N
      | dail = -18.93 deg
      | dele = -1.148 deg
      | drud = -22.97 deg
      | phi = -10 deg
      | theta = 2.793 deg
      | psi = 7.106 deg
  Angle Conversion : aerolibconvert2/Angle Conversion  IU=deg  OU=rad
  Angle Conversion1 : aerolibconvert2/Angle Conversion  IU=deg  OU=rad
  Angle Conversion2 : aerolibconvert2/Angle Conversion  IU=deg  OU=rad
  Constant : Constant  Value=0
  Constant1 : Constant  Value=0
  Mux : Mux  Inputs=3
  Signal Builder : Subsystem  Tag=STV Subsys  LoadFcn=sigbuilder_block('load');  StartFcn=sigbuilder_block('start');  StopFcn=sigbuilder_block('stop');  ClipboardFcn=sigbuilder_block('clipboard');  mask(Sigbuilder block){}
      mask help: Simulink:masks:SigbuilderBlock_MD
      mask init:
      | if ~strcmp(get_param(bdroot(gcbh),'SimulationStatus'),'stopped') tuvar = sigbuilder_block('maskInit'); end
      settings: CopyFcn=sigbuilder_block('copy');  DeleteFcn=sigbuilder_block('delete');  ModelCloseFcn=sigbuilder_block('modelClose');  PreSaveFcn=sigbuilder_block('preSave');  PauseFcn=sigbuilder_block('pause');  ContinueFcn=sigbuilder_block('continue');  NameChangeFcn=sigbuilder_block('namechange');  OpenFcn=sigbuilder_block('open',[757.5 149.25 620.25 321 ]);  CloseFcn=sigbuilder_block('close');
      mask Display: plot(0, 0, 100, 100,[2, 2, 32, 32, 2], [68, 8, 8, 68, 68],[32, 2], [38, 38], [32, 19, 2],[53, 60, 44], [32, 17, 17, 2],[16, 16, 31, 31]);txt = getActiveGroup(gcbh);text(2, 100, txt,'verticalAlignment', 'top');
  Signal Builder1 : Subsystem  Tag=STV Subsys  LoadFcn=sigbuilder_block('load');  StartFcn=sigbuilder_block('start');  StopFcn=sigbuilder_block('stop');  ClipboardFcn=sigbuilder_block('clipboard');  mask(Sigbuilder block){}
      mask help: Simulink:masks:SigbuilderBlock_MD
      mask init:
      | if ~strcmp(get_param(bdroot(gcbh),'SimulationStatus'),'stopped') tuvar = sigbuilder_block('maskInit'); end
      settings: CopyFcn=sigbuilder_block('copy');  DeleteFcn=sigbuilder_block('delete');  ModelCloseFcn=sigbuilder_block('modelClose');  PreSaveFcn=sigbuilder_block('preSave');  PauseFcn=sigbuilder_block('pause');  ContinueFcn=sigbuilder_block('continue');  NameChangeFcn=sigbuilder_block('namechange');  OpenFcn=sigbuilder_block('open',[813.75 94.5 620.25 533.25 ]);  CloseFcn=sigbuilder_block('close');
      mask Display: plot(0, 0, 100, 100,[2, 2, 32, 32, 2], [68, 8, 8, 68, 68],[32, 2], [38, 38], [32, 19, 2],[53, 60, 44], [32, 17, 17, 2],[16, 16, 31, 31]);txt = getActiveGroup(gcbh);text(2, 100, txt,'verticalAlignment', 'top');
  Sum : Sum  Inputs=++|
  Sum1 : Sum  Inputs=++|
  Sum2 : Sum  Inputs=++|
  dail_ini : Constant  Value=0
  dele_ini : Constant  Value=-1.225
  drud_ini : Constant  Value=0
  cs_command (rad) : Outport
  wires:
  Angle Conversion2/1 -> Mux/3  "drud"
  Angle Conversion1/1 -> Mux/2  "dele"
  Angle Conversion/1 -> Mux/1  "dail"
  Mux/1 -> cs_command (rad)/1
  Signal Builder/1(Signal 1) -> Sum/2
  Constant1/1 -> Sum2/2
  Constant/1 -> Sum1/2
  Sum/1 -> Angle Conversion/1
  Sum1/1 -> Angle Conversion1/1
  Sum2/1 -> Angle Conversion2/1
  dail_ini/1 -> Sum/1
  dele_ini/1 -> Sum1/1
  drud_ini/1 -> Sum2/1

== system constraints_comparison_A_4D_v2_old/Control surface input/4) Spiral ==
  Angle Conversion3 : aerolibconvert2/Angle Conversion  IU=deg  OU=rad
  Angle Conversion4 : aerolibconvert2/Angle Conversion  IU=deg  OU=rad
  Angle Conversion5 : aerolibconvert2/Angle Conversion  IU=deg  OU=rad
  Constant2 : Constant  Value=0
  Constant3 : Constant  Value=0
  Gain : Gain
  Mux : Mux  Inputs=3
  Signal Builder1 : Subsystem  Tag=STV Subsys  LoadFcn=sigbuilder_block('load');  StartFcn=sigbuilder_block('start');  StopFcn=sigbuilder_block('stop');  ClipboardFcn=sigbuilder_block('clipboard');  mask(Sigbuilder block){}
      mask help: Simulink:masks:SigbuilderBlock_MD
      mask init:
      | if ~strcmp(get_param(bdroot(gcbh),'SimulationStatus'),'stopped') tuvar = sigbuilder_block('maskInit'); end
      settings: CopyFcn=sigbuilder_block('copy');  DeleteFcn=sigbuilder_block('delete');  ModelCloseFcn=sigbuilder_block('modelClose');  PreSaveFcn=sigbuilder_block('preSave');  PauseFcn=sigbuilder_block('pause');  ContinueFcn=sigbuilder_block('continue');  NameChangeFcn=sigbuilder_block('namechange');  OpenFcn=sigbuilder_block('open',[1438.5 35.25 1428 681.75 ]);  CloseFcn=sigbuilder_block('close');
      mask Display: plot(0, 0, 100, 100,[2, 2, 32, 32, 2], [68, 8, 8, 68, 68],[32, 2], [38, 38], [32, 19, 2],[53, 60, 44], [32, 17, 17, 2],[16, 16, 31, 31]);txt = getActiveGroup(gcbh);text(2, 100, txt,'verticalAlignment', 'top');
  Sum : Sum  Inputs=++|
  Sum1 : Sum  Inputs=++|
  Sum2 : Sum  Inputs=++|
  dail_ini : Constant  Value=0
  dele_ini : Constant  Value=-1.225
  drud_ini : Constant  Value=0
  cs_command (rad) : Outport
  wires:
  Mux/1 -> cs_command (rad)/1
  Angle Conversion3/1 -> Mux/1  "dail"
  Angle Conversion4/1 -> Mux/2  "dele"
  Angle Conversion5/1 -> Mux/3  "drud"
  Signal Builder1/1(Signal 1) -> Gain/1
  Constant2/1 -> Sum/2
  Gain/1 -> Sum2/2
  Constant3/1 -> Sum1/2
  dail_ini/1 -> Sum/1
  dele_ini/1 -> Sum1/1
  drud_ini/1 -> Sum2/1
  Sum/1 -> Angle Conversion3/1
  Sum1/1 -> Angle Conversion4/1
  Sum2/1 -> Angle Conversion5/1

== system constraints_comparison_A_4D_v2_old/Control surface input/5) Dutch roll ==
  note: From the lateral_linear_model.m script:
      | The Dutch roll has a damped natural frequency of 12.9511 rad/s (2.0612 Hz)
      | So the period of the mode is: T = 1/2.0612 = 0.4852 seconds
      |
      | From simulation results:
      | T = 0.4825 seconds
      | f = 2.0725 Hz
  Angle Conversion : aerolibconvert2/Angle Conversion  IU=deg  OU=rad
  Angle Conversion1 : aerolibconvert2/Angle Conversion  IU=deg  OU=rad
  Angle Conversion2 : aerolibconvert2/Angle Conversion  IU=deg  OU=rad
  Constant : Constant  Value=0
  Constant2 : Constant  Value=0
  Gain : Gain  Commented=on  Gain=0.5
  Gain1 : Gain
  Mux : Mux  Inputs=3
  Signal Builder : Subsystem  Tag=STV Subsys  Commented=on  LoadFcn=sigbuilder_block('load');  StartFcn=sigbuilder_block('start');  StopFcn=sigbuilder_block('stop');  ClipboardFcn=sigbuilder_block('clipboard');  mask(Sigbuilder block){}
      mask help: Simulink:masks:SigbuilderBlock_MD
      mask init:
      | if ~strcmp(get_param(bdroot(gcbh),'SimulationStatus'),'stopped') tuvar = sigbuilder_block('maskInit'); end
      settings: CopyFcn=sigbuilder_block('copy');  DeleteFcn=sigbuilder_block('delete');  ModelCloseFcn=sigbuilder_block('modelClose');  PreSaveFcn=sigbuilder_block('preSave');  PauseFcn=sigbuilder_block('pause');  ContinueFcn=sigbuilder_block('continue');  NameChangeFcn=sigbuilder_block('namechange');  OpenFcn=sigbuilder_block('open',[648.75 96.75 712.5 561.75 ]);  CloseFcn=sigbuilder_block('close');
      mask Display: plot(0, 0, 100, 100,[2, 2, 32, 32, 2], [68, 8, 8, 68, 68],[32, 2], [38, 38], [32, 19, 2],[53, 60, 44], [32, 17, 17, 2],[16, 16, 31, 31]);txt = getActiveGroup(gcbh);text(2, 100, txt,'verticalAlignment', 'top');
  Signal Builder1 : Subsystem  Tag=STV Subsys  LoadFcn=sigbuilder_block('load');  StartFcn=sigbuilder_block('start');  StopFcn=sigbuilder_block('stop');  ClipboardFcn=sigbuilder_block('clipboard');  mask(Sigbuilder block){}
      mask help: Simulink:masks:SigbuilderBlock_MD
      mask init:
      | if ~strcmp(get_param(bdroot(gcbh),'SimulationStatus'),'stopped') tuvar = sigbuilder_block('maskInit'); end
      settings: CopyFcn=sigbuilder_block('copy');  DeleteFcn=sigbuilder_block('delete');  ModelCloseFcn=sigbuilder_block('modelClose');  PreSaveFcn=sigbuilder_block('preSave');  PauseFcn=sigbuilder_block('pause');  ContinueFcn=sigbuilder_block('continue');  NameChangeFcn=sigbuilder_block('namechange');  OpenFcn=sigbuilder_block('open',[386.25 30.75 718.5 675 ]);  CloseFcn=sigbuilder_block('close');
      mask Display: plot(0, 0, 100, 100,[2, 2, 32, 32, 2], [68, 8, 8, 68, 68],[32, 2], [38, 38], [32, 19, 2],[53, 60, 44], [32, 17, 17, 2],[16, 16, 31, 31]);txt = getActiveGroup(gcbh);text(2, 100, txt,'verticalAlignment', 'top');
  Signal Builder1 old (two dublets) : Subsystem  Tag=STV Subsys  LoadFcn=sigbuilder_block('load');  StartFcn=sigbuilder_block('start');  StopFcn=sigbuilder_block('stop');  ClipboardFcn=sigbuilder_block('clipboard');  mask(Sigbuilder block){}
      mask help: Simulink:masks:SigbuilderBlock_MD
      mask init:
      | if ~strcmp(get_param(bdroot(gcbh),'SimulationStatus'),'stopped') tuvar = sigbuilder_block('maskInit'); end
      settings: CopyFcn=sigbuilder_block('copy');  DeleteFcn=sigbuilder_block('delete');  ModelCloseFcn=sigbuilder_block('modelClose');  PreSaveFcn=sigbuilder_block('preSave');  PauseFcn=sigbuilder_block('pause');  ContinueFcn=sigbuilder_block('continue');  NameChangeFcn=sigbuilder_block('namechange');  OpenFcn=sigbuilder_block('open',[720.75 30.75 718.5 715.5 ]);  CloseFcn=sigbuilder_block('close');
      mask Display: plot(0, 0, 100, 100,[2, 2, 32, 32, 2], [68, 8, 8, 68, 68],[32, 2], [38, 38], [32, 19, 2],[53, 60, 44], [32, 17, 17, 2],[16, 16, 31, 31]);txt = getActiveGroup(gcbh);text(2, 100, txt,'verticalAlignment', 'top');
  Sum : Sum  Inputs=++|
  Sum1 : Sum  Inputs=++|
  Sum2 : Sum  Inputs=++|
  dail_ini : Constant  Value=0
  dele_ini : Constant  Value=-1.225
  drud_ini : Constant  Value=0
  cs_command (rad) : Outport
  wires:
  Angle Conversion2/1 -> Mux/3  "drud"
  Angle Conversion1/1 -> Mux/2  "dele"
  Angle Conversion/1 -> Mux/1  "dail"
  Mux/1 -> cs_command (rad)/1
  Signal Builder1/1(Signal 1) -> Gain1/1
  Signal Builder/1(Signal 1) -> Gain/1
  Constant/1 -> Sum/2
  Gain1/1 -> Sum2/2
  Constant2/1 -> Sum1/2
  dail_ini/1 -> Sum/1
  dele_ini/1 -> Sum1/1
  drud_ini/1 -> Sum2/1
  Sum/1 -> Angle Conversion/1
  Sum1/1 -> Angle Conversion1/1
  Sum2/1 -> Angle Conversion2/1

== system constraints_comparison_A_4D_v2_old/Subsystem14/Aerodynamics lookup ==
  Alpha (deg) : Inport
  1-D Lookup Table : Lookup_n-D  NumberOfTableDimensions=1  BreakpointsForDimension1=breakpoints1  Table=de  DiagnosticForOutOfRangeInput=Warning  InternalRulePriority=Speed  RndMeth=Simplest  InputSameDT=on
  1-D Lookup Table1 : Lookup_n-D  NumberOfTableDimensions=1  BreakpointsForDimension1=breakpoints1  Table=Cm0  DiagnosticForOutOfRangeInput=Warning  InternalRulePriority=Speed  RndMeth=Simplest  InputSameDT=on
  1-D Lookup Table2 : Lookup_n-D  NumberOfTableDimensions=1  BreakpointsForDimension1=breakpoints1  Table=Cmde  DiagnosticForOutOfRangeInput=Warning  InternalRulePriority=Speed  RndMeth=Simplest  InputSameDT=on
  1-D Lookup Table3 : Lookup_n-D  NumberOfTableDimensions=1  BreakpointsForDimension1=breakpoints1  Table=Cmq  DiagnosticForOutOfRangeInput=Warning  InternalRulePriority=Speed  RndMeth=Simplest  InputSameDT=on
  Cm0 : Outport
  Cmde : Outport  Port=2
  de_deg : Outport  Port=3
  Cmq : Outport  Port=4
  wires:
  1-D Lookup Table/1 -> de_deg/1  "de_deg"
  1-D Lookup Table1/1 -> Cm0/1  "Cm0"
  Alpha (deg)/1 -> 1-D Lookup Table3/1, 1-D Lookup Table/1, 1-D Lookup Table2/1, 1-D Lookup Table1/1  "Alpha (deg)"
  1-D Lookup Table3/1 -> Cmq/1  "Cmq"
  1-D Lookup Table2/1 -> Cmde/1  "Cmde"

== system constraints_comparison_A_4D_v2_old/Subsystem14/Compensator servo model1 ==
  Command : Inport
  Mot : Gain  Gain=K2_svo_cmp
  Saturation : Saturate  UpperLimit=max_rate_sat_cmp  LowerLimit=-max_rate_sat_cmp
  Sum : Sum  Inputs=|+-
  Sum1 : Sum  Inputs=|+-
  Svo : Gain  Gain=K1_svo_cmp
  kinematic : Subsystem
  Response : Outport
  wires:
  Sum/1 -> Svo/1
  Svo/1 -> Saturation/1
  Sum1/1 -> Mot/1
  Saturation/1 -> Sum1/1
  kinematic/1(de) -> Response/1, Sum/2
  Mot/1 -> kinematic/1(rate_dot)
  kinematic/2(de_dot) -> Sum1/2
  Command/1 -> Sum/1

== system constraints_comparison_A_4D_v2_old/Subsystem14/Compensator servo model2 ==
  Command : Inport
  Mot : Gain  Gain=K2_svo_cmp
  Saturation : Saturate  UpperLimit=max_rate_sat_cmp  LowerLimit=-max_rate_sat_cmp
  Sum : Sum  Inputs=|+-
  Sum1 : Sum  Inputs=|+-
  Svo : Gain  Gain=K1_svo_cmp
  kinematic : Subsystem
  Response : Outport
  wires:
  Command/1 -> Sum/1
  kinematic/2(de_dot) -> Sum1/2
  Mot/1 -> kinematic/1(rate_dot)
  kinematic/1(de) -> Sum/2, Response/1
  Saturation/1 -> Sum1/1
  Sum1/1 -> Mot/1
  Svo/1 -> Saturation/1
  Sum/1 -> Svo/1

== system constraints_comparison_A_4D_v2_old/Subsystem14/Compensator servo model3 ==
  Command : Inport
  Mot : Gain  Gain=K2_svo_cmp
  Saturation : Saturate  UpperLimit=max_rate_sat_cmp  LowerLimit=-max_rate_sat_cmp
  Sum : Sum  Inputs=|+-
  Sum1 : Sum  Inputs=|+-
  Svo : Gain  Gain=K1_svo_cmp
  kinematic : Subsystem
  Response : Outport
  wires:
  Sum/1 -> Svo/1
  Svo/1 -> Saturation/1
  Sum1/1 -> Mot/1
  Saturation/1 -> Sum1/1
  kinematic/1(de) -> Response/1, Sum/2
  Mot/1 -> kinematic/1(rate_dot)
  kinematic/2(de_dot) -> Sum1/2
  Command/1 -> Sum/1

== system constraints_comparison_A_4D_v2_old/Subsystem14/Compensator servo model4 ==
  Command : Inport
  Mot : Gain  Gain=K2_svo_cmp
  Saturation : Saturate  UpperLimit=max_rate_sat_cmp  LowerLimit=-max_rate_sat_cmp
  Sum : Sum  Inputs=|+-
  Sum1 : Sum  Inputs=|+-
  Svo : Gain  Gain=K1_svo_cmp
  kinematic : Subsystem
  Response : Outport
  wires:
  Command/1 -> Sum/1
  kinematic/2(de_dot) -> Sum1/2
  Mot/1 -> kinematic/1(rate_dot)
  kinematic/1(de) -> Sum/2, Response/1
  Saturation/1 -> Sum1/1
  Sum1/1 -> Mot/1
  Svo/1 -> Saturation/1
  Sum/1 -> Svo/1

== system constraints_comparison_A_4D_v2_old/Subsystem14/Extracting position vector 1 ==
  In1 : Inport
  MATLAB Function : MATLAB Function  TreatAsAtomicUnit=on
  Out1 : Outport
  wires:
  In1/1 -> MATLAB Function/1(u)
  MATLAB Function/1(y) -> Out1/1

== system constraints_comparison_A_4D_v2_old/Subsystem14/Extracting position vector 2 ==
  In1 : Inport
  MATLAB Function : MATLAB Function  TreatAsAtomicUnit=on
  Out1 : Outport
  wires:
  In1/1 -> MATLAB Function/1(u)
  MATLAB Function/1(y) -> Out1/1

== system constraints_comparison_A_4D_v2_old/Subsystem14/Extracting position vector 2  ==
  In1 : Inport
  MATLAB Function : MATLAB Function  TreatAsAtomicUnit=on
  Out1 : Outport
  wires:
  MATLAB Function/1(y) -> Out1/1
  In1/1 -> MATLAB Function/1(u)

== system constraints_comparison_A_4D_v2_old/Subsystem14/Extracting position vector 3 ==
  In1 : Inport
  MATLAB Function : MATLAB Function  TreatAsAtomicUnit=on
  Out1 : Outport
  wires:
  In1/1 -> MATLAB Function/1(u)
  MATLAB Function/1(y) -> Out1/1
